simulink model "W06_1_vrx"  (R2024b)
settings: Solver=ode4  StartTime=0.0  StopTime=inf  FixedStep=Ts_ctrl  RelTol=1e-3
values from neighbouring files (symbols this model uses):
  animate = 1    [W06_setup.m]    (also in W08_setup.m)
  center_east = 40    [W06_setup.m]    (also in W08_setup.m)
  center_north = 20    [W06_setup.m]    (also in W08_setup.m)
  crab_comp = 0    [W06_setup.m]    (also in W08_setup.m)
  F_max = 500    [W06_setup.m]    (also in W08_setup.m)
  half_beam = 1.027135    [W06_setup.m]    (also in W08_setup.m)
  k_prop = 1000 * 0.004422 * 0.2^4    (= 0.0070752)    [W06_setup.m]    (also in W08_setup.m)
  Kd_psi = 200    [W06_setup.m]    (also in W08_setup.m)
  Ki_u = 300    [W06_pid_setup.m]    (also in W06_setup.m = 100; W08_setup.m = 100)
  Kp_psi = 400    [W06_setup.m]    (also in W08_setup.m)
  Kp_u = 300    [W06_pid_setup.m]    (also in W06_setup.m; W08_setup.m)
  n_max = sqrt(F_max / k_prop)    [W06_setup.m]    (also in W08_setup.m)
  origin_east = -532    [W06_setup.m]    (also in W08_setup.m)
  origin_north = 162    [W06_setup.m]    (also in W08_setup.m)
  p_c = 0.313    [W06_setup.m]    (also in W08_setup.m)
  r_d = 25    [W06_setup.m]    (also in W08_setup.m)
  required_turns = 0    [W06_setup.m]    (also in W08_setup.m)
  tau_n = 0.30    (= 0.3)    [W06_setup.m]    (also in W08_setup.m)
  Ts_ctrl = 0.05    [W06_setup.m]    (also in W08_setup.m)
  u_ref = 1.5    [W06_setup.m]    (also in W08_setup.m)
  use_schedule = 0    [W06_setup.m]    (also in W08_setup.m)
libraries: ros2lib x5, slpidlib x1
settings Model: Creator=admin  LastModifiedBy=admin

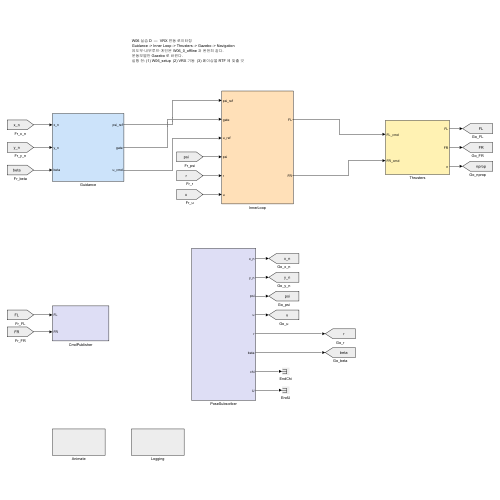
[thumbnail: Simulink's stored preview of the top-level diagram]
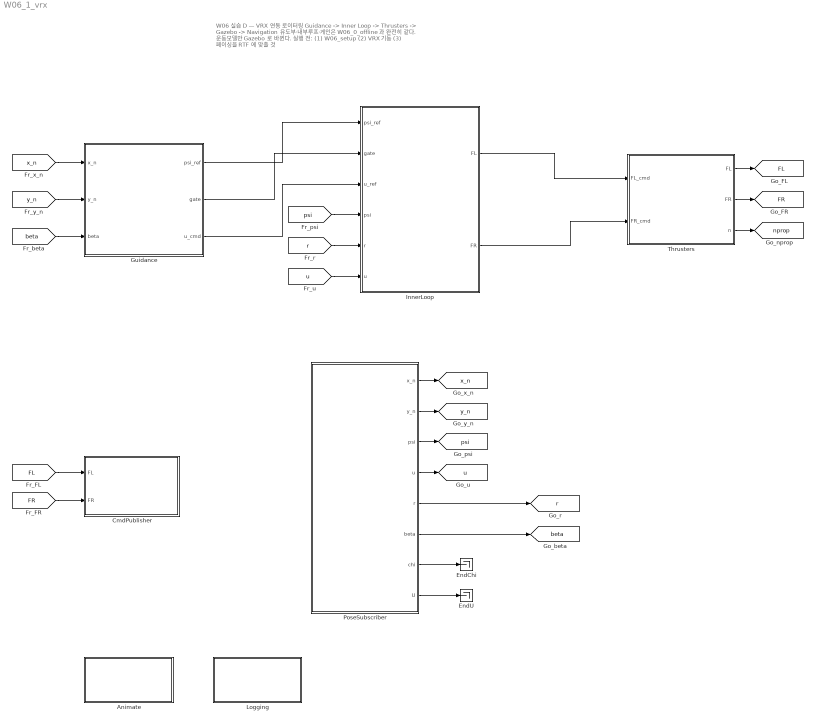
== system W06_1_vrx ==
  note: W06 실습 D  —  VRX 연동 로이터링
      | Guidance -> Inner Loop -> Thrusters -> Gazebo -> Navigation
      | 유도부·내부루프·게인은 W06_0_offline 과 완전히 같다.
      | 운동모델만 Gazebo 로 바뀐다.
      | 실행 전: (1) W06_setup  (2) VRX 기동  (3) 페이싱을 RTF 에 맞출 것
  Animate : Subsystem
  CmdPublisher : Subsystem
  EndChi : Terminator
  EndU : Terminator
  Guidance : Subsystem
  InnerLoop : Subsystem
  Logging : Subsystem
  PoseSubscriber : Subsystem
  Thrusters : Subsystem
  tag scope: FL=global, FR=global, beta=global, nprop=global, psi=global, r=global, u=global, x_n=global, y_n=global
  wires:
  PoseSubscriber/8(U) -> EndU/1
  PoseSubscriber/7(chi) -> EndChi/1
  [FR] -> CmdPublisher/2(FR)
  [FL] -> CmdPublisher/1(FL)
  InnerLoop/2(FR) -> Thrusters/2(FR_cmd)
  InnerLoop/1(FL) -> Thrusters/1(FL_cmd)
  [u] -> InnerLoop/6(u)
  [r] -> InnerLoop/5(r)
  [psi] -> InnerLoop/4(psi)
  Guidance/3(u_cmd) -> InnerLoop/3(u_ref)
  Guidance/2(gate) -> InnerLoop/2(gate)
  Guidance/1(psi_ref) -> InnerLoop/1(psi_ref)
  [beta] -> Guidance/3(beta)
  [y_n] -> Guidance/2(y_n)
  [x_n] -> Guidance/1(x_n)
  Thrusters/1(FL) -> [FL]
  Thrusters/2(FR) -> [FR]
  PoseSubscriber/6(beta) -> [beta]
  Thrusters/3(n) -> [nprop]
  PoseSubscriber/3(psi) -> [psi]
  PoseSubscriber/5(r) -> [r]
  PoseSubscriber/4(u) -> [u]
  PoseSubscriber/1(x_n) -> [x_n]
  PoseSubscriber/2(y_n) -> [y_n]

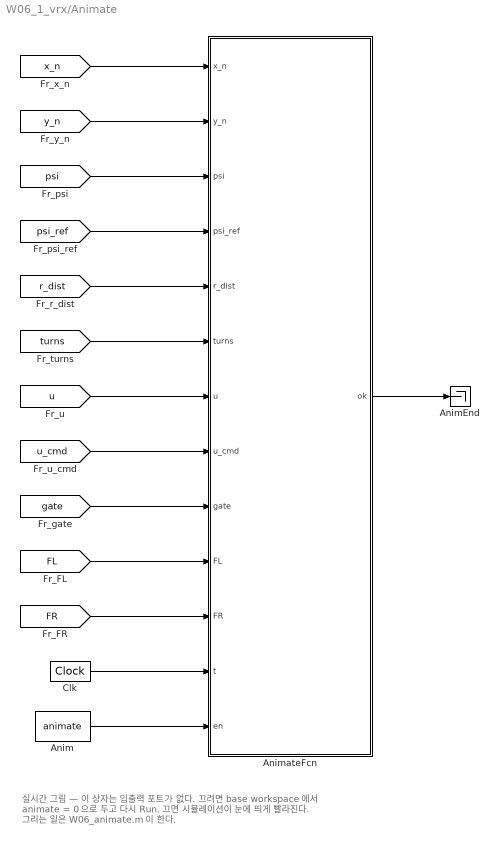
== system W06_1_vrx/Animate ==
  note: 실시간 그림 — 이 상자는 입출력 포트가 없다.
      | 끄려면 base workspace 에서  animate = 0  으로 두고 다시 Run.
      | 끄면 시뮬레이션이 눈에 띄게 빨라진다.
      | 그리는 일은 W06_animate.m 이 한다.
  Anim : Constant  Value=animate
  AnimEnd : Terminator
  AnimateFcn : MATLAB Function  TreatAsAtomicUnit=on
  Clk : DigitalClock  SampleTime=Ts_ctrl
  wires:
  [x_n] -> AnimateFcn/1(x_n)
  [y_n] -> AnimateFcn/2(y_n)
  [psi] -> AnimateFcn/3(psi)
  [psi_ref] -> AnimateFcn/4(psi_ref)
  [r_dist] -> AnimateFcn/5(r_dist)
  [turns] -> AnimateFcn/6(turns)
  [u] -> AnimateFcn/7(u)
  [u_cmd] -> AnimateFcn/8(u_cmd)
  [gate] -> AnimateFcn/9(gate)
  [FL] -> AnimateFcn/10(FL)
  [FR] -> AnimateFcn/11(FR)
  Clk/1 -> AnimateFcn/12(t)
  Anim/1 -> AnimateFcn/13(en)
  AnimateFcn/1(ok) -> AnimEnd/1

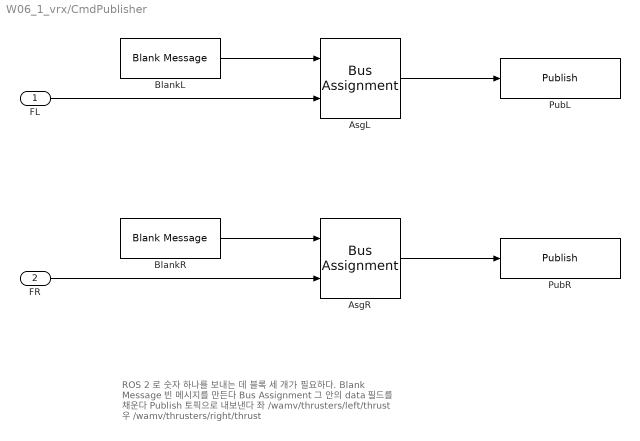
== system W06_1_vrx/CmdPublisher ==
  note: ROS 2 로 숫자 하나를 보내는 데 블록 세 개가 필요하다.
      |   Blank Message   빈 메시지를 만든다
      |   Bus Assignment  그 안의 data 필드를 채운다
      |   Publish         토픽으로 내보낸다
      |
      | 좌 /wamv/thrusters/left/thrust
      | 우 /wamv/thrusters/right/thrust
  FL : Inport
  FR : Inport  Port=2
  AsgL : BusAssignment  AssignedSignals=data
  AsgR : BusAssignment  AssignedSignals=data
  BlankL : ros2lib/Blank Message  messageClass=Message  entityType=std_msgs/Float64  messageType=std_msgs/Float64  SampleTime=Ts_ctrl
  BlankR : ros2lib/Blank Message  messageClass=Message  entityType=std_msgs/Float64  messageType=std_msgs/Float64  SampleTime=Ts_ctrl
  PubL : ros2lib/Publish  topicSource=Specify your own  topic=/wamv/thrusters/left/thrust  messageType=std_msgs/Float64  QOSHistory=Keep last  QOSDepth=1  QOSReliability=Reliable  QOSDurability=Volatile  QOSDeadline=Inf  QOSLifespan=Inf  QOSLiveliness=Automatic  QOSLeaseDuration=Inf  QOSAvoidROSNamespaceConventions=off
  PubR : ros2lib/Publish  topicSource=Specify your own  topic=/wamv/thrusters/right/thrust  messageType=std_msgs/Float64  QOSHistory=Keep last  QOSDepth=1  QOSReliability=Reliable  QOSDurability=Volatile  QOSDeadline=Inf  QOSLifespan=Inf  QOSLiveliness=Automatic  QOSLeaseDuration=Inf  QOSAvoidROSNamespaceConventions=off
  wires:
  BlankL/1 -> AsgL/1
  AsgL/1 -> PubL/1
  FL/1 -> AsgL/2
  BlankR/1 -> AsgR/1
  AsgR/1 -> PubR/1
  FR/1 -> AsgR/2

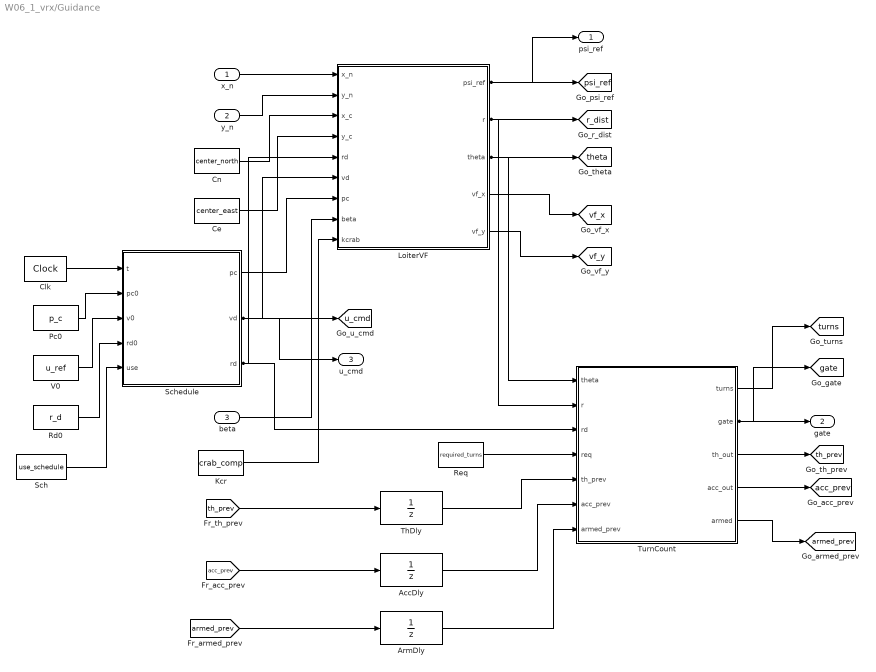
== system W06_1_vrx/Guidance ==
  x_n : Inport
  y_n : Inport  Port=2
  beta : Inport  Port=3
  AccDly : UnitDelay  Description=바퀴 수 계수기 — 표본 사이의 각 변화를 모아 감기므로 바로 앞 표본이 있어야 한다. 또한 TurnCount 가 낸 값이 TurnCount 로 되돌아와 대수 루프가 된다.  SampleTime=Ts_ctrl  HasFrameUpgradeWarning=on
  ArmDly : UnitDelay  Description=바퀴 수 계수기 — 표본 사이의 각 변화를 모아 감기므로 바로 앞 표본이 있어야 한다. 또한 TurnCount 가 낸 값이 TurnCount 로 되돌아와 대수 루프가 된다.  SampleTime=Ts_ctrl  HasFrameUpgradeWarning=on
  Ce : Constant  Value=center_east
  Clk : DigitalClock  SampleTime=Ts_ctrl
  Cn : Constant  Value=center_north
  Kcr : Constant  Value=crab_comp
  LoiterVF : MATLAB Function  TreatAsAtomicUnit=on
  Pc0 : Constant  Value=p_c
  Rd0 : Constant  Value=r_d
  Req : Constant  Value=required_turns
  Sch : Constant  Value=use_schedule
  Schedule : MATLAB Function  TreatAsAtomicUnit=on
  ThDly : UnitDelay  Description=바퀴 수 계수기 — 표본 사이의 각 변화를 모아 감기므로 바로 앞 표본이 있어야 한다. 또한 TurnCount 가 낸 값이 TurnCount 로 되돌아와 대수 루프가 된다.  SampleTime=Ts_ctrl  HasFrameUpgradeWarning=on
  TurnCount : MATLAB Function  TreatAsAtomicUnit=on
  V0 : Constant  Value=u_ref
  psi_ref : Outport
  gate : Outport  Port=2
  u_cmd : Outport  Port=3
  tag scope: acc_prev=global, armed_prev=global, gate=global, psi_ref=global, r_dist=global, th_prev=global, theta=global, turns=global, u_cmd=global, vf_x=global, vf_y=global
  wires:
  Cn/1 -> LoiterVF/3(x_c)
  Clk/1 -> Schedule/1(t)
  ArmDly/1 -> TurnCount/7(armed_prev)
  Pc0/1 -> Schedule/2(pc0)
  V0/1 -> Schedule/3(v0)
  Rd0/1 -> Schedule/4(rd0)
  Sch/1 -> Schedule/5(use)
  y_n/1 -> LoiterVF/2(y_n)
  x_n/1 -> LoiterVF/1(x_n)
  Ce/1 -> LoiterVF/4(y_c)
  Schedule/1(pc) -> LoiterVF/7(pc)
  TurnCount/5(armed) -> [armed_prev]
  Schedule/2(vd) -> LoiterVF/6(vd), u_cmd/1, [u_cmd]
  LoiterVF/4(vf_x) -> [vf_x]
  Schedule/3(rd) -> TurnCount/3(rd), LoiterVF/5(rd)
  beta/1 -> LoiterVF/8(beta)
  Kcr/1 -> LoiterVF/9(kcrab)
  [th_prev] -> ThDly/1
  [acc_prev] -> AccDly/1
  Req/1 -> TurnCount/4(req)
  [armed_prev] -> ArmDly/1
  LoiterVF/1(psi_ref) -> psi_ref/1, [psi_ref]
  TurnCount/3(th_out) -> [th_prev]
  ThDly/1 -> TurnCount/5(th_prev)
  LoiterVF/2(r) -> TurnCount/2(r), [r_dist]
  LoiterVF/3(theta) -> [theta], TurnCount/1(theta)
  LoiterVF/5(vf_y) -> [vf_y]
  AccDly/1 -> TurnCount/6(acc_prev)
  TurnCount/1(turns) -> [turns]
  TurnCount/2(gate) -> gate/1, [gate]
  TurnCount/4(acc_out) -> [acc_prev]

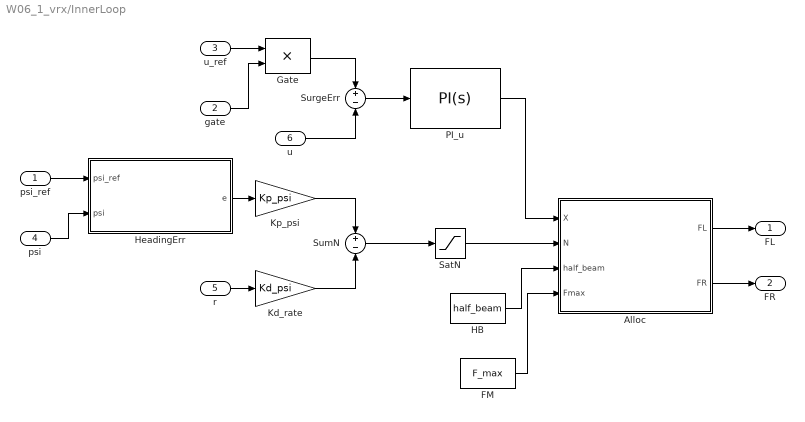
== system W06_1_vrx/InnerLoop ==
  psi_ref : Inport
  gate : Inport  Port=2
  u_ref : Inport  Port=3
  psi : Inport  Port=4
  r : Inport  Port=5
  u : Inport  Port=6
  Alloc : MATLAB Function  TreatAsAtomicUnit=on
  FM : Constant  Value=F_max
  Gate : Product
  HB : Constant  Value=half_beam
  HeadingErr : MATLAB Function  TreatAsAtomicUnit=on
  Kd_rate : Gain  Gain=Kd_psi
  Kp_psi : Gain  Gain=Kp_psi
  PI_u : slpidlib/PID Controller  Controller=PI  Form=Parallel  TimeDomain=Continuous-time  UseExternalTs=off  SampleTime=-1  IntegratorMethod=Forward Euler  FilterMethod=Forward Euler  ControllerParametersSource=internal  P=Kp_u  I=Ki_u  UseKiTs=off  D=0  UseExternalDerivativeSource=off  N=100  UseFilter=on  TunerSelectOption=Transfer Function Based (PID Tuner App)  InitialConditionSource=internal  InitialConditionForIntegrator=0  InitialConditionForFilter=0  DifferentiatorICPrevScaledInput=0  ExternalReset=none  TrackingMode=off  Kt=1  LimitOutput=on  SatLimitsSource=internal  UpperSaturationLimit=2*F_max  LowerSaturationLimit=-2*F_max  LinearizeAsGain=on  AntiWindupMode=clamping  Kb=1  LimitIntegrator=off  UpperIntegratorSaturationLimit=inf  LowerIntegratorSaturationLimit=-inf  POutMin=[]  POutMax=[]  IOutMin=[]  IOutMax=[]  DOutMin=[]  DOutMax=[]  NOutMin=[]  NOutMax=[]  SumOutMin=[]  SumOutMax=[]  SaturationOutMin=[]  SaturationOutMax=[]  PParamMin=[]  PParamMax=[]  IParamMin=[]  IParamMax=[]  DParamMin=[]  DParamMax=[]  NParamMin=[]  NParamMax=[]  KbParamMin=[]  KbParamMax=[]  KtParamMin=[]  KtParamMax=[]  KbOutMin=[]  KbOutMax=[]  KtOutMin=[]  KtOutMax=[]  IntegratorOutMin=[]  IntegratorOutMax=[]  FilterOutMin=[]  FilterOutMax=[]  SumI1OutMin=[]  SumI1OutMax=[]  SumI2OutMin=[]  SumI2OutMax=[]  SumI3OutMin=[]  SumI3OutMax=[]  SumI4OutMin=[]  SumI4OutMax=[]  SumDOutMin=[]  SumDOutMax=[]  DifferentiatorOutMin=[]  DifferentiatorOutMax=[]  FilterDiffOutCoefMin=[]  FilterDiffOutCoefMax=[]  ReciprocalOutMin=[]  ReciprocalOutMax=[]  SumDenOutMin=[]  SumDenOutMax=[]  SumNumOutMin=[]  SumNumOutMax=[]  DivideOutMin=[]  DivideOutMax=[]  UdiffTsProdOutMin=[]  UdiffTsProdOutMax=[]  NTsProdOutMin=[]  NTsProdOutMax=[]  UintegralTsProdOutMin=[]  UintegralTsProdOutMax=[]  UngainTsProdOutMin=[]  UngainTsProdOutMax=[]  ClampingZeroOutDataTypeStr=Inherit: Inherit via back propagation  ClampingZeroOutMin=[]  ClampingZeroOutMax=[]  FilterDenConstantOutDataTypeStr=Inherit: Inherit via back propagation  FilterDenConstantOutMin=[]  FilterDenConstantOutMax=[]  PCopyOutDataTypeStr=Inherit: Inherit via back propagation  PCopyOutMin=[]  PCopyOutMax=[]  NCopyOutDataTypeStr=Inherit: Inherit via back propagation  NCopyOutMin=[]  NCopyOutMax=[]  IntegratorContinuousStateAttributes=''  IntegratorStateMustResolveToSignalObject=off  IntegratorRTWStateStorageClass=Auto  FilterContinuousStateAttributes=''  FilterStateMustResolveToSignalObject=off  FilterRTWStateStorageClass=Auto  ParallelPVariant=InternalParameters  IdealPVariant=Disabled  IVariant=InternalParameters  DVariant=Disabled  IntegratorVariant=Continuous  SatVariant=Enabled  AWVariant=ContClampingParallel  PCopyVariant=Disabled  TRVariant=Disabled  FdbkBlocksVariant=Forward  IdealPFdbkVariant=Disabled  SatFdbkVariant=Disabled  DerivativeFilterVariant=Disabled  NVariant=Disabled  NCopyVariant=Disabled_SignalSpec  FilterICVariant=Disabled  IntegratorICVariant=InternalICs  ExternalResetVariant=Disabled  TRSumVariant=Passthrough  SumFdbkVariant=Disabled  SumVariant=Sum_PI  TsampFilterVariant=InternalTs  TsampNgainVariant=Passthrough  TsampIntegralVariant=Disabled_SignalSpec  ExternalSaturationOutDataTypeStr=Inherit: Same as second input  DerivativeSourceVariant=Disabled  PreIntVariant=InternalPreInt
  SatN : Saturate  UpperLimit=2*F_max*half_beam  LowerLimit=-2*F_max*half_beam
  SumN : Sum  Inputs=+-
  SurgeErr : Sum  Inputs=+-
  FL : Outport
  FR : Outport  Port=2
  wires:
  HeadingErr/1(e) -> Kp_psi/1
  psi_ref/1 -> HeadingErr/1(psi_ref)
  Kd_rate/1 -> SumN/2
  psi/1 -> HeadingErr/2(psi)
  u_ref/1 -> Gate/1
  gate/1 -> Gate/2
  u/1 -> SurgeErr/2
  Gate/1 -> SurgeErr/1
  r/1 -> Kd_rate/1
  Kp_psi/1 -> SumN/1
  SurgeErr/1 -> PI_u/1
  SumN/1 -> SatN/1
  FM/1 -> Alloc/4(Fmax)
  PI_u/1 -> Alloc/1(X)
  SatN/1 -> Alloc/2(N)
  HB/1 -> Alloc/3(half_beam)
  Alloc/1(FL) -> FL/1
  Alloc/2(FR) -> FR/1

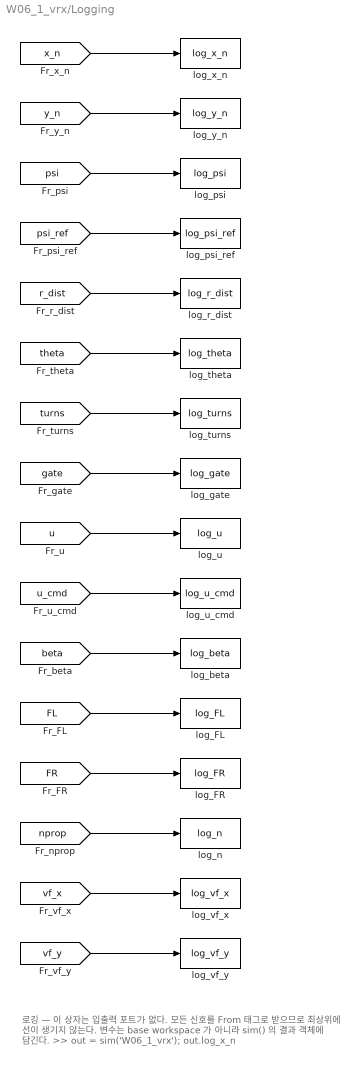
== system W06_1_vrx/Logging ==
  note: 로깅 — 이 상자는 입출력 포트가 없다.
      | 모든 신호를 From 태그로 받으므로 최상위에 선이 생기지 않는다.
      | 변수는 base workspace 가 아니라 sim() 의 결과 객체에 담긴다.
      |   >> out = sim('W06_1_vrx');  out.log_x_n
  log_FL : ToWorkspace  VariableName=log_FL  SaveFormat=Timeseries  SampleTime=Ts_ctrl
  log_FR : ToWorkspace  VariableName=log_FR  SaveFormat=Timeseries  SampleTime=Ts_ctrl
  log_beta : ToWorkspace  VariableName=log_beta  SaveFormat=Timeseries  SampleTime=Ts_ctrl
  log_gate : ToWorkspace  VariableName=log_gate  SaveFormat=Timeseries  SampleTime=Ts_ctrl
  log_n : ToWorkspace  VariableName=log_n  SaveFormat=Timeseries  SampleTime=Ts_ctrl
  log_psi : ToWorkspace  VariableName=log_psi  SaveFormat=Timeseries  SampleTime=Ts_ctrl
  log_psi_ref : ToWorkspace  VariableName=log_psi_ref  SaveFormat=Timeseries  SampleTime=Ts_ctrl
  log_r_dist : ToWorkspace  VariableName=log_r_dist  SaveFormat=Timeseries  SampleTime=Ts_ctrl
  log_theta : ToWorkspace  VariableName=log_theta  SaveFormat=Timeseries  SampleTime=Ts_ctrl
  log_turns : ToWorkspace  VariableName=log_turns  SaveFormat=Timeseries  SampleTime=Ts_ctrl
  log_u : ToWorkspace  VariableName=log_u  SaveFormat=Timeseries  SampleTime=Ts_ctrl
  log_u_cmd : ToWorkspace  VariableName=log_u_cmd  SaveFormat=Timeseries  SampleTime=Ts_ctrl
  log_vf_x : ToWorkspace  VariableName=log_vf_x  SaveFormat=Timeseries  SampleTime=Ts_ctrl
  log_vf_y : ToWorkspace  VariableName=log_vf_y  SaveFormat=Timeseries  SampleTime=Ts_ctrl
  log_x_n : ToWorkspace  VariableName=log_x_n  SaveFormat=Timeseries  SampleTime=Ts_ctrl
  log_y_n : ToWorkspace  VariableName=log_y_n  SaveFormat=Timeseries  SampleTime=Ts_ctrl
  wires:
  [x_n] -> log_x_n/1
  [y_n] -> log_y_n/1
  [psi] -> log_psi/1
  [psi_ref] -> log_psi_ref/1
  [r_dist] -> log_r_dist/1
  [theta] -> log_theta/1
  [turns] -> log_turns/1
  [gate] -> log_gate/1
  [u] -> log_u/1
  [u_cmd] -> log_u_cmd/1
  [beta] -> log_beta/1
  [FL] -> log_FL/1
  [FR] -> log_FR/1
  [nprop] -> log_n/1
  [vf_x] -> log_vf_x/1
  [vf_y] -> log_vf_y/1

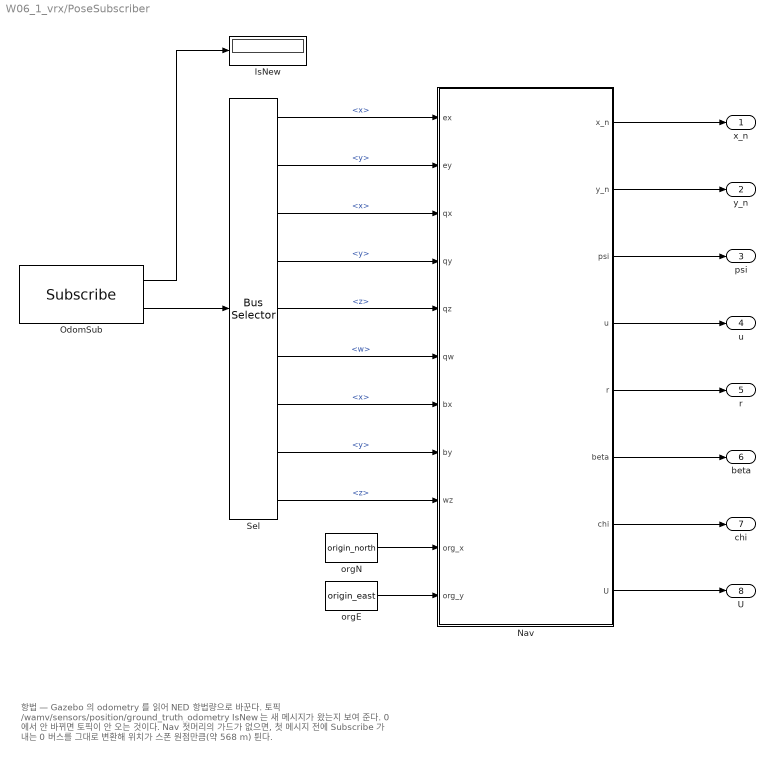
== system W06_1_vrx/PoseSubscriber ==
  note: 항법 — Gazebo 의 odometry 를 읽어 NED 항법량으로 바꾼다.
      |   토픽 /wamv/sensors/position/ground_truth_odometry
      |
      | IsNew 는 새 메시지가 왔는지 보여 준다. 0 에서 안 바뀌면 토픽이 안 오는 것이다.
      | Nav 첫머리의 가드가 없으면, 첫 메시지 전에 Subscribe 가 내는 0 버스를
      | 그대로 변환해 위치가 스폰 원점만큼(약 568 m) 튄다.
  IsNew : Display
  Nav : MATLAB Function  TreatAsAtomicUnit=on
  OdomSub : ros2lib/Subscribe  topicSource=Specify your own  topic=/wamv/sensors/position/ground_truth_odometry  messageType=nav_msgs/Odometry  sampleTime=Ts_ctrl  QOSHistory=Keep last  QOSDepth=1  QOSReliability=Reliable  QOSDurability=Volatile  QOSDeadline=Inf  QOSLifespan=Inf  QOSLiveliness=Automatic  QOSLeaseDuration=Inf  QOSAvoidROSNamespaceConventions=off
  Sel : BusSelector  OutputSignals=pose.pose.position.x,pose.pose.position.y,pose.pose.orientation.x,pose.pose.orientation.y,pose.pose.orientation.z,pose.pose.orientation.w,twist.twist.linear.x,twist.twist.linear.y,twist.twist.angular.z
  orgE : Constant  Value=origin_east
  orgN : Constant  Value=origin_north
  x_n : Outport
  y_n : Outport  Port=2
  psi : Outport  Port=3
  u : Outport  Port=4
  r : Outport  Port=5
  beta : Outport  Port=6
  chi : Outport  Port=7
  U : Outport  Port=8
  wires:
  OdomSub/1 -> IsNew/1
  OdomSub/2 -> Sel/1
  Sel/1 -> Nav/1(ex)  "<x>"
  Sel/2 -> Nav/2(ey)  "<y>"
  Sel/3 -> Nav/3(qx)  "<x>"
  Sel/4 -> Nav/4(qy)  "<y>"
  Sel/5 -> Nav/5(qz)  "<z>"
  Sel/6 -> Nav/6(qw)  "<w>"
  Sel/7 -> Nav/7(bx)  "<x>"
  Sel/8 -> Nav/8(by)  "<y>"
  Sel/9 -> Nav/9(wz)  "<z>"
  orgN/1 -> Nav/10(org_x)
  orgE/1 -> Nav/11(org_y)
  Nav/1(x_n) -> x_n/1
  Nav/2(y_n) -> y_n/1
  Nav/3(psi) -> psi/1
  Nav/4(u) -> u/1
  Nav/5(r) -> r/1
  Nav/6(beta) -> beta/1
  Nav/7(chi) -> chi/1
  Nav/8(U) -> U/1

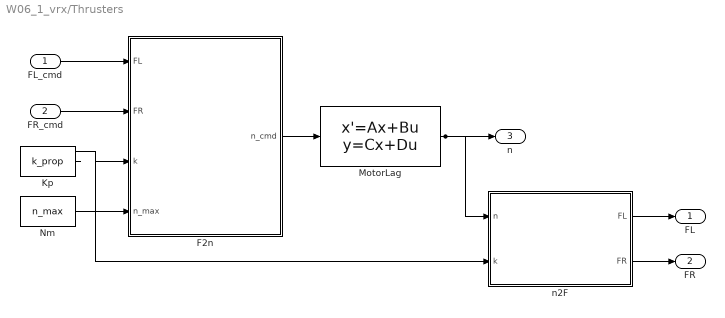
== system W06_1_vrx/Thrusters ==
  FL_cmd : Inport
  FR_cmd : Inport  Port=2
  F2n : MATLAB Function  TreatAsAtomicUnit=on
  Kp : Constant  Value=k_prop
  MotorLag : StateSpace  A=-eye(2)/tau_n  B=eye(2)/tau_n  C=eye(2)  D=zeros(2)  InitialCondition=zeros(2,1)
  Nm : Constant  Value=n_max
  n2F : MATLAB Function  TreatAsAtomicUnit=on
  FL : Outport
  FR : Outport  Port=2
  n : Outport  Port=3
  wires:
  n2F/2(FR) -> FR/1
  FL_cmd/1 -> F2n/1(FL)
  FR_cmd/1 -> F2n/2(FR)
  n2F/1(FL) -> FL/1
  MotorLag/1 -> n2F/1(n), n/1
  Kp/1 -> n2F/2(k), F2n/3(k)
  Nm/1 -> F2n/4(n_max)
  F2n/1(n_cmd) -> MotorLag/1

== matlab function W06_1_vrx/Thrusters/n2F ==
  data: n input; FL output; k input; FR output
function [FL, FR] = n2F(n, k)
%#codegen
% Forward propeller law. Thrust is quadratic in shaft speed.
FL = k * n(1) * abs(n(1));
FR = k * n(2) * abs(n(2));

== matlab function W06_1_vrx/PoseSubscriber/Nav ==
  data: ex input; x_n output; ey input; qx input; qy input; qz input; qw input; bx input; by input; wz input; org_x input; org_y input; y_n output; psi output; u output; r output; beta output; chi output; U output
function [x_n, y_n, psi, u, r, beta, chi, U] = Nav(ex, ey, qx, qy, qz, qw, bx, by, wz, org_x, org_y)
%#codegen
% Gazebo/ROS uses ENU with a body frame of x-forward, y-LEFT, z-UP.
% Marine control uses NED with x-forward, y-STARBOARD, z-DOWN.
% 첫 메시지가 도착하기 전에는 Subscribe 가 0 으로 채운 버스를 낸다.
% 그대로 쓰면 위치가 스폰 원점만큼(약 568 m) 튀어 로그 첫 점이 망가진다.
if ex == 0 && ey == 0
    x_n = 0; y_n = 0; psi = 0; u = 0; r = 0; beta = 0; chi = 0; U = 0;
    return
end
x_n = ey - org_x;
y_n = ex - org_y;
yaw_enu = atan2(2*(qw*qz + qx*qy), 1 - 2*(qy*qy + qz*qz));
p   = pi/2 - yaw_enu;
psi = atan2(sin(p), cos(p));
u = bx;
v = -by;
r = -wz;
U    = sqrt(u*u + v*v);
beta = atan2(v, u);
c    = psi + beta;
chi  = atan2(sin(c), cos(c));

== matlab function W06_1_vrx/Animate/AnimateFcn ==
  data: x_n input; y_n input; psi input; psi_ref input; r_dist input; turns input; u input; ok output; u_cmd input; gate input; FL input; FR input; t input; en input
function ok = AnimateFcn(x_n, y_n, psi, psi_ref, r_dist, turns, u, u_cmd, gate, FL, FR, t, en)
%#codegen
% Live plot while the model runs. A MATLAB Function block cannot
% plot, so the drawing function is declared extrinsic: Simulink
% calls plain MATLAB instead of generating code for it.
coder.extrinsic('W06_animate');
ok = 1;
if en > 0.5
    W06_animate(x_n, y_n, psi, psi_ref, r_dist, turns, u, u_cmd, gate, FL, FR, t);
end

== matlab function W06_1_vrx/Guidance/LoiterVF ==
  data: x_n input; psi_ref output; y_n input; x_c input; y_c input; rd input; vd input; pc input; beta input; kcrab input; r output; theta output; vf_x output; vf_y output
function [psi_ref, r, theta, vf_x, vf_y] = LoiterVF(x_n, y_n, x_c, y_c, rd, vd, pc, beta, kcrab)
%#codegen
% Circular-orbit vector field guidance.
%   Jung, Lim, Lee, Bang, "Unmanned Aircraft Vector Field Path Following
%   with Arrival Angle Control", eq. (9) and (13).
%
%   rd  desired orbit radius [m]
%   vd  desired speed [m/s]
%   pc  shaping parameter.  SIGN sets the turn direction:
%         pc > 0  clockwise,   pc < 0  counter-clockwise
%       A smaller |pc| pulls the vehicle harder onto the circle.

dx = x_n - x_c;
dy = y_n - y_c;

r     = sqrt(dx*dx + dy*dy);      % distance from the centre
theta = atan2(dy, dx);            % bearing of the vehicle from centre
if r < 1e-6, r = 1e-6; end        % the centre itself is singular

% eq. (9): the field written in polar components
N = sqrt((r - rd)^2 + (pc*r)^2);
if N < 1e-9, N = 1e-9; end
r_dot   = -vd * (r - rd) / N;     % radial     : closes the gap
rth_dot =  vd * pc * r   / N;     % tangential : goes round

% polar -> NED. The magnitude of this vector is always vd.
vf_x = r_dot*cos(theta) - rth_dot*sin(theta);
vf_y = r_dot*sin(theta) + rth_dot*cos(theta);

% eq. (13): the field gives a COURSE, i.e. a velocity direction.
% The boat can only be told a HEADING. In a turn the two differ by
% the crab angle beta, and that difference shows up as a radius error.
%   kcrab = 0  command the field angle directly (the paper form)
%   kcrab = 1  subtract beta so the VELOCITY lines up with the field
chi_d   = atan2(vf_y, vf_x);
p       = chi_d - kcrab*beta;
psi_ref = atan2(sin(p), cos(p));

== matlab function W06_1_vrx/Guidance/Schedule ==
  data: t input; pc output; pc0 input; v0 input; rd0 input; use input; vd output; rd output
function [pc, vd, rd] = Schedule(t, pc0, v0, rd0, use)
%#codegen
% Change the loiter direction, speed and radius while the model runs.
% Direction is set by the SIGN of pc, speed by vd, radius by rd.
if use < 0.5
    pc = pc0;   vd = v0;       rd = rd0;
elseif t < 150
    pc = pc0;   vd = v0;       rd = rd0;        % as configured
elseif t < 300
    pc = -pc0;  vd = v0;       rd = rd0;        % reverse direction
elseif t < 450
    pc = -pc0;  vd = v0*1.6;   rd = rd0;        % faster
else
    pc = -pc0;  vd = v0*1.6;   rd = rd0*0.6;    % tighter circle
end

== matlab function W06_1_vrx/Guidance/TurnCount ==
  data: theta input; turns output; r input; rd input; req input; th_prev input; acc_prev input; armed_prev input; gate output; th_out output; acc_out output; armed output
function [turns, gate, th_out, acc_out, armed] = TurnCount( ...
         theta, r, rd, req, th_prev, acc_prev, armed_prev)
%#codegen
% Count how many times the boat has gone round, then stop it.
% Same idea as calculate_turns in the UGV Stateflow example: start
% counting only after the boat has actually reached the circle,
% otherwise the approach leg would be counted as part of a lap.

tol = 0.3*rd;                     % "on the circle": steady radius error is p_c*v*tau (up to ~7 m at p_c = 1), so the band must be wider than that
th_out = theta;

if armed_prev < 0.5
    acc_out = 0;
    if abs(r - rd) <= tol
        armed = 1;                % reached the circle, start counting
    else
        armed = 0;
    end
else
    armed = 1;
    d = theta - th_prev;
    d = atan2(sin(d), cos(d));    % wrap: +pi to -pi must not count
    acc_out = acc_prev + d;
end

turns = abs(acc_out) / (2*pi);

% req = 0 means keep going forever
if (req > 0) && (turns >= req)
    gate = 0;                     % mission done, stop the boat
else
    gate = 1;
end

== matlab function W06_1_vrx/InnerLoop/HeadingErr ==
  data: psi_ref input; e output; psi input
function e = HeadingErr(psi_ref, psi)
%#codegen
% Shortest signed angle, wrapped to [-pi, pi).
d = psi_ref - psi;
e = atan2(sin(d), cos(d));

== matlab function W06_1_vrx/InnerLoop/Alloc ==
  data: X input; FL output; N input; half_beam input; Fmax input; FR output
function [FL, FR] = Alloc(X, N, half_beam, Fmax)
%#codegen
% Differential thrust allocation for two aft thrusters.
FL = X/2 + N/(2*half_beam);
FR = X/2 - N/(2*half_beam);
if FL >  Fmax, FL =  Fmax; end
if FL < -Fmax, FL = -Fmax; end
if FR >  Fmax, FR =  Fmax; end
if FR < -Fmax, FR = -Fmax; end

== matlab function W06_1_vrx/Thrusters/F2n ==
  data: FL input; n_cmd output; FR input; k input; n_max input
function n_cmd = F2n(FL, FR, k, n_max)
%#codegen
% Inverse propeller law:  F = k*n*|n|  ->  n = sign(F)*sqrt(|F|/k)
F = [FL; FR];
n_cmd = zeros(2,1);
for i = 1:2
    ni = sign(F(i)) * sqrt(abs(F(i))/k);
    if ni >  n_max, ni =  n_max; end
    if ni < -n_max, ni = -n_max; end
    n_cmd(i) = ni;
end
